simulink model "Battery_modelling_thevenin_model"  (R2025a)
settings: Solver=FixedStepAuto  StartTime=0.0  StopTime=200  FixedStep=Ts  RelTol=1e-3
values from neighbouring files (symbols this model uses):
  C1 = 2000    [Battery_parameters.m]
  Ct = 4800    [Battery_parameters.m]    (also in EV_parameters.m = 3)
  I = 2    [Battery_parameters.m]
  OCV = 8    [Battery_parameters.m]
  R1 = 0.09    [Battery_parameters.m]
  Ro = 0.07    [Battery_parameters.m]    (also in EV_parameters.m = 0.03)
  v1 = 0.5    [Battery_parameters.m]
undefined symbols (not defined in the file or in its folder): DiscIntNeverNeededParam, SOC_i
settings Model: Creator=91944  LastModifiedBy=91944

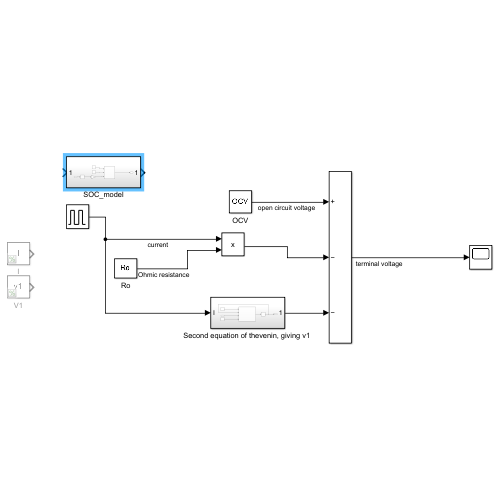
[thumbnail: Simulink's stored preview of the top-level diagram]
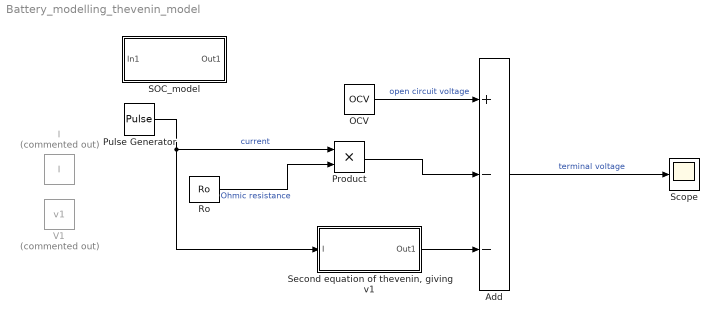
== system Battery_modelling_thevenin_model ==
  Add : Sum  Inputs=+--
  I : Constant  Commented=on  Value=I  SampleTime=-1
  OCV : Constant  Value=OCV  SampleTime=-1
  Product : Product
  Pulse Generator : DiscretePulseGenerator  PulseType=Time based  Amplitude=2  Period=200  PulseWidth=5  PhaseDelay=15
  Ro : Constant  Value=Ro  SampleTime=-1
  SOC_model : Subsystem
  Scope : Scope
      settings: ActiveDisplayYMinimum=7.385278617492987  ActiveDisplayYMaximum=8.4481562042844889
  "Second equation of thevenin, giving v1 " : Subsystem
  V1 : Constant  Commented=on  Value=v1  SampleTime=-1
  wires:
  Pulse Generator/1 -> "Second equation of thevenin, giving v1 "/1(I), Product/1  "current"
  Ro/1 -> Product/2  "Ohmic resistance"
  Product/1 -> Add/2
  OCV/1 -> Add/1  "open circuit voltage"
  Add/1 -> Scope/1  "terminal voltage"
  "Second equation of thevenin, giving v1 "/1(Out1) -> Add/3

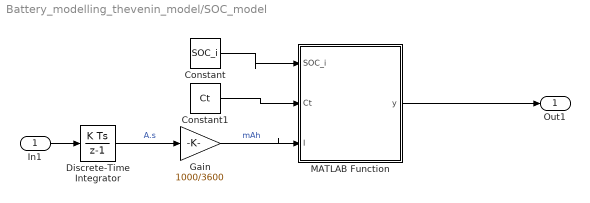
== system Battery_modelling_thevenin_model/SOC_model ==
  In1 : Inport
  Constant : Constant  Value=SOC_i
  Constant1 : Constant  Value=Ct
  Discrete-Time Integrator : DiscreteIntegrator  SampleTime=-1  ICPrevOutput=DiscIntNeverNeededParam  ICPrevScaledInput=DiscIntNeverNeededParam
  Gain : Gain  Gain=1000/3600
  MATLAB Function : MATLAB Function  TreatAsAtomicUnit=on
  Out1 : Outport
  wires:
  In1/1 -> Discrete-Time Integrator/1
  Discrete-Time Integrator/1 -> Gain/1  "A.s"
  MATLAB Function/1(y) -> Out1/1
  Constant/1 -> MATLAB Function/1(SOC_i)
  Constant1/1 -> MATLAB Function/2(Ct)
  Gain/1 -> MATLAB Function/3(I)  "mAh"

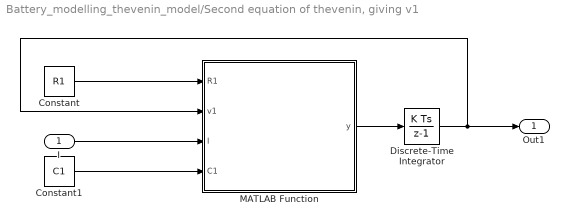
== system Battery_modelling_thevenin_model/Second equation of thevenin, giving v1  ==
  I : Inport
  Constant : Constant  Value=R1  SampleTime=-1
  Constant1 : Constant  Value=C1  SampleTime=-1
  Discrete-Time Integrator : DiscreteIntegrator  SampleTime=-1  ICPrevOutput=DiscIntNeverNeededParam  ICPrevScaledInput=DiscIntNeverNeededParam
  MATLAB Function : MATLAB Function  TreatAsAtomicUnit=on
  Out1 : Outport
  wires:
  I/1 -> MATLAB Function/3(I)
  MATLAB Function/1(y) -> Discrete-Time Integrator/1
  Constant/1 -> MATLAB Function/1(R1)
  Constant1/1 -> MATLAB Function/4(C1)
  Discrete-Time Integrator/1 -> MATLAB Function/2(v1), Out1/1

== matlab function Battery_modelling_thevenin_model/SOC_model/MATLAB Function ==
  data: SOC_i input; y output; Ct input; I input
function y = fcn(SOC_i,Ct,I)

y = SOC_i-100*I/Ct; % 100 to change from percentage

== matlab function Battery_modelling_thevenin_model/Second equation of thevenin, giving v1 /MATLAB Function ==
  data: R1 input; y output; v1 input; I input; C1 input
function y = fcn(R1,v1,I,C1)
y = -v1/(R1*C1)+I/C1 ;
